simulink model "EKF_InverseDynamic_2dof_pole"  (R2023b)
settings: Solver=VariableStepAuto  StartTime=0.0  StopTime=Tend_slk  RelTol=1e-3
values from neighbouring files (symbols this model uses):
  g = 9.81    [EKF_main_inverse_2dof_pole.m]
  IMU_a_b_bias = ones(3,1)*0.1    [EKF_main_inverse_2dof_pole.m]
  IMU_a_b_variance = IMU_var_bias_matrix(:,1)    [EKF_main_inverse_2dof_pole.m]
  IMU_mf_b_bias = ones(3,1)*0.1    [EKF_main_inverse_2dof_pole.m]
  IMU_mf_b_variance = IMU_var_bias_matrix(:,4)    [EKF_main_inverse_2dof_pole.m]
  IMU_w_b_bias = IMU_var_bias_matrix(:,2)    [EKF_main_inverse_2dof_pole.m]
  IMU_w_b_variance = IMU_var_bias_matrix(:,3)    [EKF_main_inverse_2dof_pole.m]
  mf = [22602; 0; -42062;]    [EKF_main_inverse_2dof_pole.m]
  P0 = diag([P0_ph_meas,P0_th_meas,P0_ps_meas,P0_bias_wp,P0_bias_wq,P0_bias_wr])    [EKF_main_inverse_2dof_pole.m]
  param = [Ixx;Iyy;Izz;l;k1;k2;k3;k4;b;m]    [EKF_main_inverse_2dof_pole.m]
  Q = diag([q_angle,q_angle,q_angle, q_bias_w_b,q_bias_w_b,q_bias_w_b])    [EKF_main_inverse_2dof_pole.m]
  R = diag([r_th_meas,r_th_meas,r_ps_meas])    [EKF_main_inverse_2dof_pole.m]
  Ts_EKF_integr = 0.01    [EKF_main_inverse_2dof_pole.m]
  Ts_EKF_meas = 0.05    [EKF_main_inverse_2dof_pole.m]
  Ts_slk = 0.01    [EKF_main_inverse_2dof_pole.m]
  x0 = [1;1;1;0;0;0]*0.01    [EKF_main_inverse_2dof_pole.m]
  x0EKF = [ph0;th0;ps0;bias_wp0;bias_wq0;bias_wr0]    [EKF_main_inverse_2dof_pole.m]
undefined symbols (not defined in the file or in its folder): Kpole, x_eq
libraries: simulink x3
settings Model: Creator=teoma  LastModifiedBy=asus

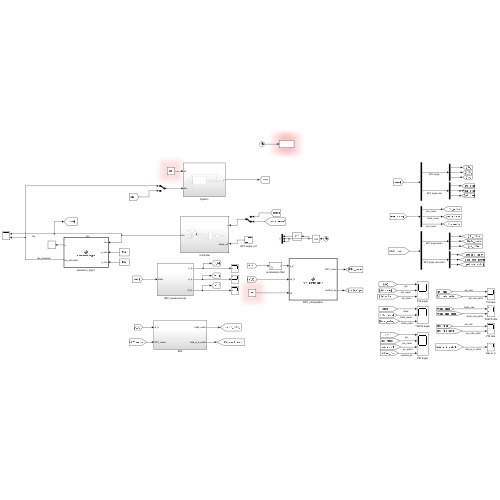
[thumbnail: Simulink's stored preview of the top-level diagram]
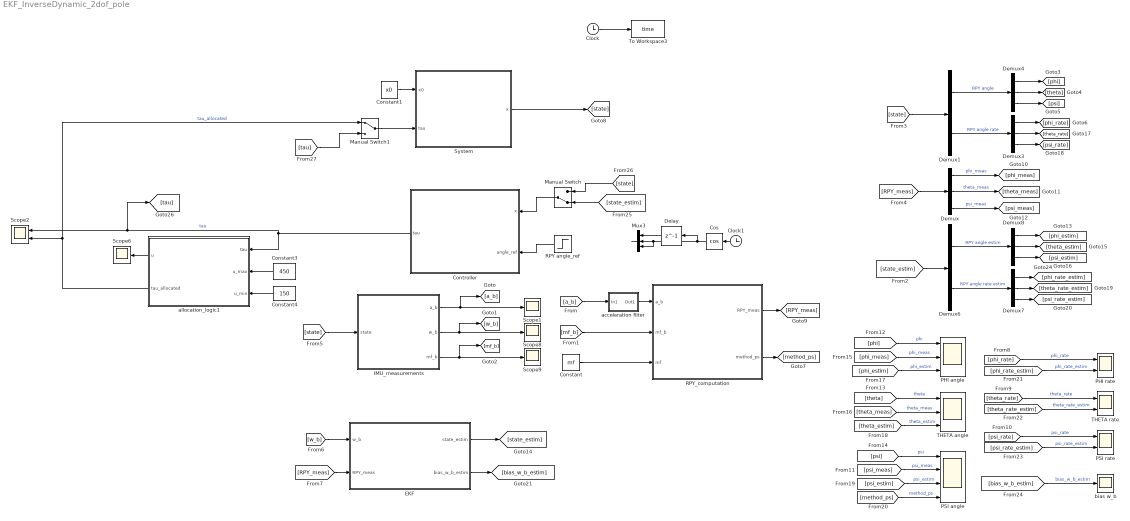
== system EKF_InverseDynamic_2dof_pole ==
  Clock : Clock
  Clock1 : Clock
  Constant : Constant  Value=mf
  Constant1 : Constant  Value=x0
  Constant3 : Constant  Value=450  SampleTime=0.01
  Constant4 : Constant  Value=150  SampleTime=0.01
  Controller : Subsystem
  Cos : Trigonometry  Operator=cos
  Delay : Delay  DelayLength=1  SampleTime=0.01
  Demux{,3..4,7..8} (5 alike) : Demux  Outputs=3
  Demux1 : Demux  Outputs=2
  Demux6 : Demux  Outputs=2
  EKF : Subsystem
  IMU_measurements : Subsystem
  Manual Switch : ManualSwitch  CurrentSetting=0
  Manual Switch1 : ManualSwitch
  Mux3 : Mux  Inputs=3
  PHI angle : Scope  NumInputPorts=3
  PHI rate : Scope  NumInputPorts=2
  PSI angle : Scope  NumInputPorts=4
  PSI rate : Scope  NumInputPorts=2
  RPY angle_ref : Step  Time=20  After=[0.52;0.52]  SampleTime=0
  RPY_computation : MATLAB Function  TreatAsAtomicUnit=on
  Scope{1,6,8..9} (4 alike) : Scope
  Scope2 : Scope  NumInputPorts=2
  System : Subsystem
  THETA angle : Scope  NumInputPorts=3
  THETA rate : Scope  NumInputPorts=2
  To Workspace3 : ToWorkspace  VariableName=time  SampleTime=Ts_slk
      settings: Save2DSignal=2-D array (concatenate along first dimension)
  acceleration filter : Subsystem  mask{p=5}
      mask prompts: p "pole"
  allocation_logic1 : MATLAB Function  TreatAsAtomicUnit=on
  bias w_b : Scope
  wires:
  Demux4/3 -> [psi]
  Demux4/2 -> [theta]
  Constant1/1 -> System/1(x0)
  Demux1/2 -> Demux3/1  "RPY angle rate"
  System/1(x) -> [state]
  Demux4/1 -> [phi]
  Clock/1 -> To Workspace3/1
  Demux1/1 -> Demux4/1  "RPY angle"
  IMU_measurements/1(a_b) -> [a_b], Scope1/1
  IMU_measurements/2(w_b) -> Scope8/1, [w_b]
  IMU_measurements/3(mf_b) -> [mf_b], Scope9/1
  [a_b] -> acceleration filter/1(In1)
  [mf_b] -> RPY_computation/2(mf_b)
  Constant/1 -> RPY_computation/3(mf)
  RPY_computation/1(RPY_meas) -> [RPY_meas]
  [state] -> IMU_measurements/1(state)
  [w_b] -> EKF/1(w_b)
  [RPY_meas] -> EKF/2(RPY_meas)
  [phi] -> PHI angle/1  "phi"
  [phi_meas] -> PHI angle/2  "phi_meas"
  [phi_estim] -> PHI angle/3  "phi_estim"
  [theta] -> THETA angle/1  "theta"
  [theta_meas] -> THETA angle/2  "theta_meas"
  [theta_estim] -> THETA angle/3  "theta_estim"
  [psi] -> PSI angle/1  "psi"
  [psi_meas] -> PSI angle/2  "psi_meas"
  [psi_estim] -> PSI angle/3  "psi_estim"
  RPY_computation/2(method_ps) -> [method_ps]
  acceleration filter/1(Out1) -> RPY_computation/1(a_b)
  EKF/1(state_estim) -> [state_estim]
  EKF/2(bias_w_b_estim) -> [bias_w_b_estim]
  [method_ps] -> PSI angle/4  "method_ps"
  [state] -> Demux1/1
  Demux3/3 -> [psi_rate]
  Demux3/1 -> [phi_rate]
  Demux3/2 -> [theta_rate]
  [RPY_meas] -> Demux/1
  Demux/2 -> [theta_meas]  "theta_meas"
  Demux/3 -> [psi_meas]  "psi_meas"
  Demux/1 -> [phi_meas]  "phi_meas"
  Demux7/1 -> [phi_rate_estim]
  [state_estim] -> Demux6/1
  Demux8/1 -> [phi_estim]
  Demux8/2 -> [theta_estim]
  Demux7/2 -> [theta_rate_estim]
  Demux6/2 -> Demux7/1  "RPY angle rate estim"
  Demux7/3 -> [psi_rate_estim]
  Demux8/3 -> [psi_estim]
  Demux6/1 -> Demux8/1  "RPY angle estim"
  [phi_rate] -> PHI rate/1  "phi_rate"
  [phi_rate_estim] -> PHI rate/2  "phi_rate_estim"
  [psi_rate] -> PSI rate/1  "psi_rate"
  [psi_rate_estim] -> PSI rate/2  "psi_rate_estim"
  [theta_rate] -> THETA rate/1  "theta_rate"
  [theta_rate_estim] -> THETA rate/2  "theta_rate_estim"
  [bias_w_b_estim] -> bias w_b/1  "bias_w_b_estim"
  [state_estim] -> Manual Switch/2
  Clock1/1 -> Cos/1
  Cos/1 -> Mux3/2, Mux3/3, Delay/1
  Delay/1 -> Mux3/1
  Mux3/1 -> ?
  RPY angle_ref/1 -> Controller/2(angle_ref)
  Manual Switch/1 -> Controller/1(x)
  [state] -> Manual Switch/1
  Manual Switch1/1 -> System/2("tau ")
  [tau] -> Manual Switch1/2
  allocation_logic1/1(u) -> Scope6/1
  Controller/1(tau) -> Scope2/1, [tau], allocation_logic1/1(tau)  "tau"
  allocation_logic1/2(tau_allocated) -> Manual Switch1/1, Scope2/2  "tau_allocated"
  Constant3/1 -> allocation_logic1/2(u_max)
  Constant4/1 -> allocation_logic1/3(u_min)

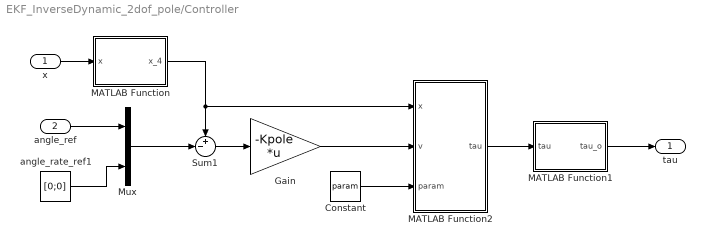
== system EKF_InverseDynamic_2dof_pole/Controller ==
  x : Inport
  angle_ref : Inport  Port=2
  Constant : Constant  Value=param
  Gain : Gain  Gain=-Kpole  Multiplication=Matrix(K*u) (u vector)
  MATLAB Function : MATLAB Function  TreatAsAtomicUnit=on
  MATLAB Function1 : MATLAB Function  TreatAsAtomicUnit=on
  MATLAB Function2 : MATLAB Function  TreatAsAtomicUnit=on
  Mux : Mux  Inputs=2
  Sum1 : Sum  Inputs=+-|
  angle_rate_ref1 : Constant  Value=[0;0]
  tau : Outport
  wires:
  angle_rate_ref1/1 -> Mux/2
  Mux/1 -> Sum1/2
  Constant/1 -> MATLAB Function2/3(param)
  Gain/1 -> MATLAB Function2/2(v)
  MATLAB Function2/1(tau) -> MATLAB Function1/1(tau)
  MATLAB Function/1(x_4) -> MATLAB Function2/1(x), Sum1/1
  angle_ref/1 -> Mux/1
  Sum1/1 -> Gain/1
  MATLAB Function1/1(tau_o) -> tau/1
  x/1 -> MATLAB Function/1(x)

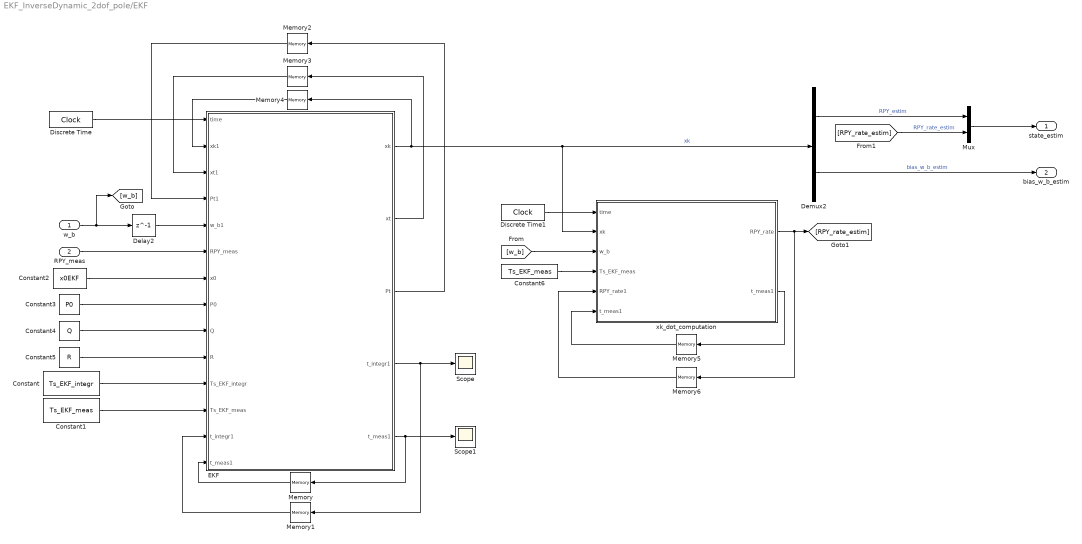
== system EKF_InverseDynamic_2dof_pole/EKF ==
  w_b : Inport
  RPY_meas : Inport  Port=2
  Constant : Constant  Value=Ts_EKF_integr
  Constant1 : Constant  Value=Ts_EKF_meas
  Constant2 : Constant  Value=x0EKF
  Constant3 : Constant  Value=P0
  Constant4 : Constant  Value=Q
  Constant5 : Constant  Value=R
  Constant6 : Constant  Value=Ts_EKF_meas
  Delay2 : Delay  DelayLength=1  SampleTime=Ts_EKF_integr
  Demux2 : Demux  Outputs=2
  Discrete Time : DigitalClock  SampleTime=Ts_slk
  Discrete Time1 : DigitalClock  SampleTime=Ts_slk
  EKF : MATLAB Function  TreatAsAtomicUnit=on
  Memory{,1..6} (7 alike) : Memory
  Mux : Mux  Inputs=2
  Scope : Scope
  Scope1 : Scope
  xk_dot_computation : MATLAB Function  TreatAsAtomicUnit=on
  state_estim : Outport
  bias_w_b_estim : Outport  Port=2
  wires:
  w_b/1 -> Delay2/1, [w_b]
  Constant4/1 -> EKF/9(Q)
  Constant2/1 -> EKF/7(x0)
  Constant5/1 -> EKF/10(R)
  Memory/1 -> EKF/14("t_meas1 ")
  EKF/2(xt) -> Memory3/1
  Memory2/1 -> EKF/4(Pt1)
  EKF/3(Pt) -> Memory2/1
  RPY_meas/1 -> EKF/6(RPY_meas)
  Discrete Time/1 -> EKF/1(time)
  Memory3/1 -> EKF/3(xt1)
  Memory1/1 -> EKF/13("t_integr1 ")
  Constant3/1 -> EKF/8(P0)
  EKF/5(t_meas1) -> Scope1/1, Memory/1
  EKF/4(t_integr1) -> Scope/1, Memory1/1
  Delay2/1 -> EKF/5(w_b1)
  Constant/1 -> EKF/11(Ts_EKF_integr)
  Constant1/1 -> EKF/12(Ts_EKF_meas)
  Memory4/1 -> EKF/2(xk1)
  xk_dot_computation/2(t_meas1) -> Memory5/1
  Memory5/1 -> xk_dot_computation/6("t_meas1 ")
  Memory6/1 -> xk_dot_computation/5(RPY_rate1)
  xk_dot_computation/1(RPY_rate) -> [RPY_rate_estim], Memory6/1
  [w_b] -> xk_dot_computation/3(w_b)
  Discrete Time1/1 -> xk_dot_computation/1(time)
  Demux2/2 -> bias_w_b_estim/1  "bias_w_b_estim"
  Demux2/1 -> Mux/1  "RPY_estim"
  EKF/1(xk) -> xk_dot_computation/2(xk), Demux2/1, Memory4/1  "xk"
  [RPY_rate_estim] -> Mux/2  "RPY_rate_estim"
  Mux/1 -> state_estim/1
  Constant6/1 -> xk_dot_computation/4(Ts_EKF_meas)

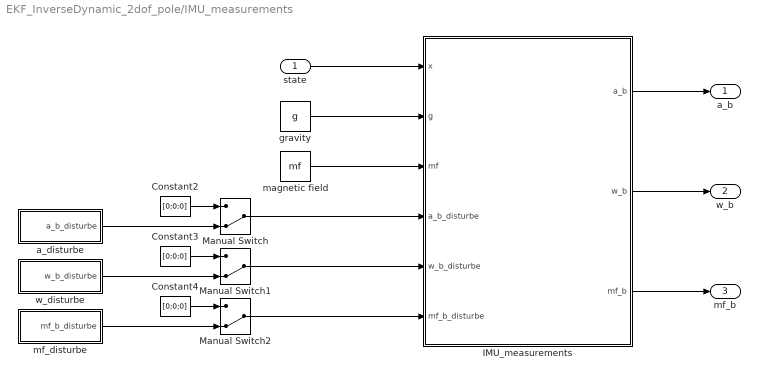
== system EKF_InverseDynamic_2dof_pole/IMU_measurements ==
  state : Inport
  Constant2 : Constant  Value=[0;0;0]
  Constant3 : Constant  Value=[0;0;0]
  Constant4 : Constant  Value=[0;0;0]
  IMU_measurements : MATLAB Function  TreatAsAtomicUnit=on
  Manual Switch : ManualSwitch  CurrentSetting=0
  Manual Switch1 : ManualSwitch  CurrentSetting=0
  Manual Switch2 : ManualSwitch  CurrentSetting=0
  a_disturbe : Subsystem  mask{on_off_bias=on bias, on_off_variance=on variance}
      mask prompts: on_off_bias "on-off bias"; on_off_variance "on-off variance"
  gravity : Constant  Value=g
  magnetic field : Constant  Value=mf
  mf_disturbe : Subsystem  mask{on_off_bias=on bias, on_off_variance=on variance}
      mask prompts: on_off_bias "on-off bias"; on_off_variance "on-off variance"
  w_disturbe : Subsystem  mask{on_off_bias=on bias, on_off_variance=on variance}
      mask prompts: on_off_bias "on-off bias"; on_off_variance "on-off variance"
  a_b : Outport
  w_b : Outport  Port=2
  mf_b : Outport  Port=3
  wires:
  state/1 -> IMU_measurements/1(x)
  gravity/1 -> IMU_measurements/2(g)
  magnetic field/1 -> IMU_measurements/3(mf)
  a_disturbe/1(a_b_disturbe) -> Manual Switch/2
  w_disturbe/1(w_b_disturbe) -> Manual Switch1/2
  mf_disturbe/1(mf_b_disturbe) -> Manual Switch2/2
  IMU_measurements/1(a_b) -> a_b/1
  IMU_measurements/2(w_b) -> w_b/1
  IMU_measurements/3(mf_b) -> mf_b/1
  Constant2/1 -> Manual Switch/1
  Constant3/1 -> Manual Switch1/1
  Constant4/1 -> Manual Switch2/1
  Manual Switch2/1 -> IMU_measurements/6(mf_b_disturbe)
  Manual Switch1/1 -> IMU_measurements/5(w_b_disturbe)
  Manual Switch/1 -> IMU_measurements/4(a_b_disturbe)

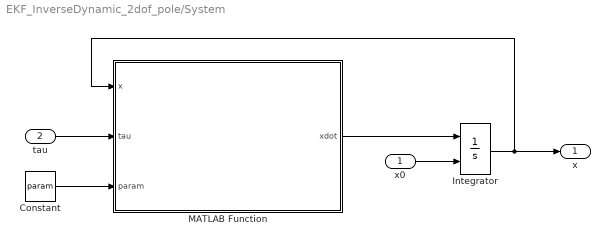
== system EKF_InverseDynamic_2dof_pole/System ==
  x0 : Inport
  "tau " : Inport  Port=2
  Constant : Constant  Value=param
  Integrator : Integrator  InitialConditionSource=external  InitialCondition=x_eq
  MATLAB Function : MATLAB Function  TreatAsAtomicUnit=on
  x : Outport
  wires:
  Integrator/1 -> MATLAB Function/1(x), x/1
  MATLAB Function/1(xdot) -> Integrator/1
  "tau "/1 -> MATLAB Function/2(tau)
  Constant/1 -> MATLAB Function/3(param)
  x0/1 -> Integrator/2

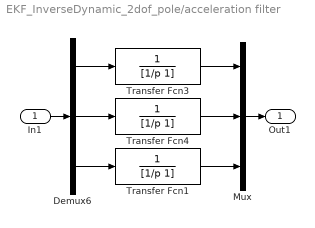
== system EKF_InverseDynamic_2dof_pole/acceleration filter ==
  In1 : Inport
  Demux6 : Demux  Outputs=3
  Mux : Mux  Inputs=3
  Transfer Fcn1 : TransferFcn  Denominator=[1/p 1]
  Transfer Fcn3 : TransferFcn  Denominator=[1/p 1]
  Transfer Fcn4 : TransferFcn  Denominator=[1/p 1]
  Out1 : Outport
  wires:
  Transfer Fcn4/1 -> Mux/2
  Demux6/3 -> Transfer Fcn1/1
  Mux/1 -> Out1/1
  Transfer Fcn1/1 -> Mux/3
  Transfer Fcn3/1 -> Mux/1
  In1/1 -> Demux6/1
  Demux6/1 -> Transfer Fcn3/1
  Demux6/2 -> Transfer Fcn4/1

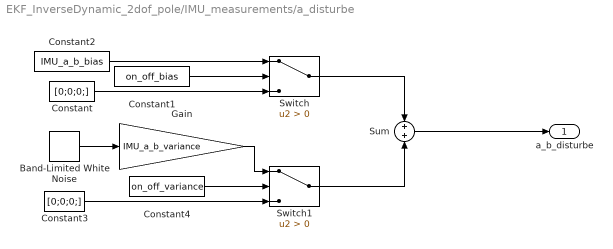
== system EKF_InverseDynamic_2dof_pole/IMU_measurements/a_disturbe ==
  Band-Limited White Noise : simulink/Sources/Band-Limited White Noise  Cov=[1]  Ts=0.1  seed=[23341]
  Constant : Constant  Value=[0;0;0;]
  Constant1 : Constant  Value=on_off_bias
  Constant2 : Constant  Value=IMU_a_b_bias
  Constant3 : Constant  Value=[0;0;0;]
  Constant4 : Constant  Value=on_off_variance
  Gain : Gain  Gain=IMU_a_b_variance
  Sum : Sum  Inputs=+|+
  Switch : Switch  Criteria=u2 > Threshold  SaturateOnIntegerOverflow=off  InputSameDT=off
  Switch1 : Switch  Criteria=u2 > Threshold  SaturateOnIntegerOverflow=off  InputSameDT=off
  a_b_disturbe : Outport
  wires:
  Constant2/1 -> Switch/1
  Sum/1 -> a_b_disturbe/1
  Constant/1 -> Switch/3
  Constant1/1 -> Switch/2
  Band-Limited White Noise/1 -> Gain/1
  Gain/1 -> Switch1/1
  Constant3/1 -> Switch1/3
  Constant4/1 -> Switch1/2
  Switch/1 -> Sum/1
  Switch1/1 -> Sum/2

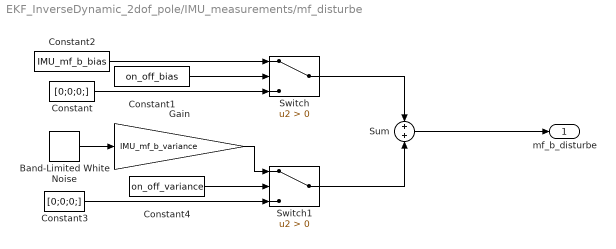
== system EKF_InverseDynamic_2dof_pole/IMU_measurements/mf_disturbe ==
  Band-Limited White Noise : simulink/Sources/Band-Limited White Noise  Cov=[1]  Ts=0.1  seed=[23341]
  Constant : Constant  Value=[0;0;0;]
  Constant1 : Constant  Value=on_off_bias
  Constant2 : Constant  Value=IMU_mf_b_bias
  Constant3 : Constant  Value=[0;0;0;]
  Constant4 : Constant  Value=on_off_variance
  Gain : Gain  Gain=IMU_mf_b_variance
  Sum : Sum  Inputs=+|+
  Switch : Switch  Criteria=u2 > Threshold  SaturateOnIntegerOverflow=off  InputSameDT=off
  Switch1 : Switch  Criteria=u2 > Threshold  SaturateOnIntegerOverflow=off  InputSameDT=off
  mf_b_disturbe : Outport
  wires:
  Constant2/1 -> Switch/1
  Sum/1 -> mf_b_disturbe/1
  Constant/1 -> Switch/3
  Constant1/1 -> Switch/2
  Band-Limited White Noise/1 -> Gain/1
  Gain/1 -> Switch1/1
  Constant3/1 -> Switch1/3
  Constant4/1 -> Switch1/2
  Switch/1 -> Sum/1
  Switch1/1 -> Sum/2

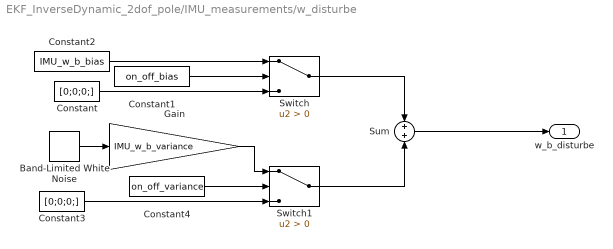
== system EKF_InverseDynamic_2dof_pole/IMU_measurements/w_disturbe ==
  Band-Limited White Noise : simulink/Sources/Band-Limited White Noise  Cov=[1]  Ts=0.1  seed=[23341]
  Constant : Constant  Value=[0;0;0;]
  Constant1 : Constant  Value=on_off_bias
  Constant2 : Constant  Value=IMU_w_b_bias
  Constant3 : Constant  Value=[0;0;0;]
  Constant4 : Constant  Value=on_off_variance
  Gain : Gain  Gain=IMU_w_b_variance
  Sum : Sum  Inputs=+|+
  Switch : Switch  Criteria=u2 > Threshold  SaturateOnIntegerOverflow=off  InputSameDT=off
  Switch1 : Switch  Criteria=u2 > Threshold  SaturateOnIntegerOverflow=off  InputSameDT=off
  w_b_disturbe : Outport
  wires:
  Constant2/1 -> Switch/1
  Sum/1 -> w_b_disturbe/1
  Constant/1 -> Switch/3
  Constant1/1 -> Switch/2
  Band-Limited White Noise/1 -> Gain/1
  Gain/1 -> Switch1/1
  Constant3/1 -> Switch1/3
  Constant4/1 -> Switch1/2
  Switch/1 -> Sum/1
  Switch1/1 -> Sum/2

== matlab function EKF_InverseDynamic_2dof_pole/Controller/MATLAB Function1 ==
  data: tau input; tau_o output
function tau_o=fcn(tau)
% Inputs:   tau    (torque 2x1)         
%
% Outputs:  tau_o  (torque 3x1)

% States in input
tau_1     =       tau(1,1);     %  roll torque
tau_2     =       tau(2,1);     %  pitch torque
 


% States in output
tau_o      =       zeros(3,1);
tau_o(1,1) =       tau_1;   
tau_o(2,1) =       tau_2;
tau_o(3,1) =       0;

== matlab function EKF_InverseDynamic_2dof_pole/Controller/MATLAB Function2 ==
  data: x input; v input; tau output; param input
function tau = fcn(x,v,param)
% Inputs:
%           x       (model state)
%           v       (new input to the feedback system)           
%           param   (model parameters)
%
% Outputs:  tau     (torque)

% Parameters
g        =       9.81;           %  gravity acceleration (m/s^2)
Ixx      =       param(1,1);     %  moment of inertia 
Iyy      =       param(2,1);     %  moment of inertia
Izz      =       param(3,1);     %  moment of inertia 

% States
phi      =       x(1,1);     %  roll angle (rad)
theta    =       x(2,1);     %  pitch angle (rad)
phi_dot  =       x(3,1);     %  roll rate (rad/s)
theta_dot=       x(4,1);     %  pitch rate (rad/s)

cph         =       cos(phi);
cth         =       cos(theta);
sph         =       sin(phi);
sth         =       sin(theta);

% Coriolis matrix
C11=  0;
C12= (Iyy)*(theta_dot*cph*sph);
C21= (Iyy)*(theta_dot*cph*sph);
C22= 0;

C  = [C11 C12;
      C21 C22];

% Inertia matrix
J11= Ixx;
J12= 0;
J21= 0;
J22= Iyy*cph^2;

J  = [J11 J12;
     J21 J22];

%% Control law
tau = zeros(2,1);
tau = J*v+C*x(3:4,1);

== matlab function EKF_InverseDynamic_2dof_pole/allocation_logic1 ==
  data: tau input; u_max input; u output; tau_allocated output; u_min input; param parameter
function [u, tau_allocated] = allocation_logic(tau,u_max,u_min,param)
% Allocation Logic Block: computes the corresponding control command
% u = [u1,u2,u3,u4] given the torque command tau = [tau_phi, tau_theta, tau_phi]

% control command limits
%%u_min = 100;
% u_max = 1000;

l  = param(4,1);
k1 = param(5,1);
k2 = param(6,1);
k3 = param(7,1);
k4 = param(8,1);
b  = param(9,1);

u = zeros(4,1);
% [tau_ph; tau_th; tau_ps] = Mtau_u * [u1;u2;u3;u4]
Mtau_u = [0       0        l*k3    -l*k4;
         -l*k1    l*k2     0        0;
         -b      -b        b        b;];
% Minv = Mtau_u'*inv(Mtau_u*Mtau_u');
% up = Minv*tau;
% un = zeros(4,1);
% if min(up(:)) < u_min 
%     un = ones(4,1)*(u_min - min(up(:)));
% end
% u = up+un;
% for i = 1:1:4
%     if u(i,1) > u_max
%         u(i,1) = u_max;
%     end
% end
if tau(1) >= 0
    u(4) = u_min;
    u(3) = (tau(1) + l*k4*u(4))/(l*k3);
else
    u(3) = u_min;
    u(4) = (-tau(1) + l*k3*u(3))/(l*k4);
end
if tau(2) >= 0
    u(1) = u_min;
    u(2) = (tau(2) + l*k1*u(1))/(l*k2);
else
    u(2) = u_min;
    u(1) = (-tau(2) + l*k2*u(2))/(l*k1);
end
u = min(u_max,u);
tau_allocated = Mtau_u*u;

== matlab function EKF_InverseDynamic_2dof_pole/Controller/MATLAB Function ==
  data: x input; x_4 output
function x_4=fcn(x)
% Inputs:   x      (model state 6x1)         
%
% Outputs:  x_4  (model state 4x1)

% States in input
phi      =       x(1,1);     %  roll angle (rad)
theta    =       x(2,1);     %  pitch angle (rad)
psi      =       x(3,1);     %  yaw angle (rad)  
phi_dot  =       x(4,1);     %  roll rate (rad/s)
theta_dot=       x(5,1);     %  pitch rate (rad/s)
psi_dot  =       x(6,1);     %  yaw rate (rad/s)  


% States in output
x_4      =       zeros(4,1);
x_4(1,1) =       phi;   
x_4(2,1) =       theta;
x_4(3,1) =       phi_dot;
x_4(4,1) =       theta_dot;

== matlab function EKF_InverseDynamic_2dof_pole/System/MATLAB Function ==
  data: x input; tau input; xdot output; param input
function xdot=quadcopter(x,tau,param)
% Inputs:
%           x       (model state)
%           tau     (torque)           
%           param   (model parameters)
%
% Outputs:  x_dot  (derivative of the state with respect to time)

% Parameters
g        =       9.81;           %  gravity acceleration (m/s^2)
Ixx      =       param(1,1);     %  moment of inertia 
Iyy      =       param(2,1);     %  moment of inertia
Izz      =       param(3,1);     %  moment of inertia 

% States
phi      =       x(1,1);     %  roll angle (rad)
theta    =       x(2,1);     %  pitch angle (rad)
psi      =       x(3,1);     %  yaw angle (rad)  
phi_dot  =       x(4,1);     %  roll rate (rad/s)
theta_dot=       x(5,1);     %  pitch rate (rad/s)
psi_dot  =       x(6,1);     %  yaw rate (rad/s)  

cph         =       cos(phi);
cth         =       cos(theta);
cps         =       cos(psi);
sph         =       sin(phi);
sth         =       sin(theta);
sps         =       sin(psi);  

% Coriolis matrix
C11=  0;
C12= (Iyy-Izz)*(theta_dot*cph*sph+psi_dot*sph^2*cth)+(Izz-Iyy)*psi_dot*cph^2*cth-Ixx*psi_dot*cth;
C13= (Izz-Iyy)*psi_dot*cph*sph*cth^2;
C21= (Izz-Iyy)*(theta_dot*cph*sph+psi_dot*sph*cth)+(Iyy-Izz)*psi_dot*cph^2*cth+Ixx*psi_dot*cth;
C22= (Izz-Iyy)*psi_dot*cph*sph;
C23= -Ixx*psi_dot*sth*cth+Iyy*psi_dot*sph^2*sth*cth+Izz*psi_dot*cph^2*sth*cth;
C31= (Iyy-Izz)*psi_dot*cth^2*sph*cph-Ixx*theta_dot*cth;
C32= (Izz-Iyy)*(theta_dot*cph*sph*sth+phi_dot*sph^2*cth)+(Iyy-Izz)*phi_dot*cph^2*cth+Ixx*psi_dot*sth*cth-Iyy*psi_dot*sph^2*sth*cth-Izz*psi_dot*cph^2*sth*cth;
C33= (Iyy-Izz)*phi_dot*cph*sph*cth^2-Iyy*theta_dot*sph^2*cth*sth-Izz*theta_dot*cph^2*cth*sth+Ixx*theta_dot*cth*sth;

C  = [C11 C12 C13;
    C21 C22 C23;
    C31 C32 C33];

% Inertia matrix
J11= Ixx;
J12= 0;
J13= -Ixx*sth;
J21= 0;
J22= Iyy*cph^2+Izz*sph^2;
J23= (Iyy-Izz)*cph*sph*cth;
J31= -Ixx*sth;
J32= (Iyy-Izz)*cph*sph*cth;
J33= Ixx*sth^2+Iyy*sph^2*cth^2+Izz*cph^2*cth^2;

J  = [J11 J12 J13;
    J21 J22 J23;
    J31 J32 J33];
%% Model equations
invJ = [ (J22*J33 - J23*J32)/(J11*J22*J33 - J11*J23*J32 - J12*J21*J33 + J12*J23*J31 + J13*J21*J32 - J13*J22*J31), -(J12*J33 - J13*J32)/(J11*J22*J33 - J11*J23*J32 - J12*J21*J33 + J12*J23*J31 + J13*J21*J32 - J13*J22*J31),  (J12*J23 - J13*J22)/(J11*J22*J33 - J11*J23*J32 - J12*J21*J33 + J12*J23*J31 + J13*J21*J32 - J13*J22*J31);
         -(J21*J33 - J23*J31)/(J11*J22*J33 - J11*J23*J32 - J12*J21*J33 + J12*J23*J31 + J13*J21*J32 - J13*J22*J31),  (J11*J33 - J13*J31)/(J11*J22*J33 - J11*J23*J32 - J12*J21*J33 + J12*J23*J31 + J13*J21*J32 - J13*J22*J31), -(J11*J23 - J13*J21)/(J11*J22*J33 - J11*J23*J32 - J12*J21*J33 + J12*J23*J31 + J13*J21*J32 - J13*J22*J31);
         (J21*J32 - J22*J31)/(J11*J22*J33 - J11*J23*J32 - J12*J21*J33 + J12*J23*J31 + J13*J21*J32 - J13*J22*J31), -(J11*J32 - J12*J31)/(J11*J22*J33 - J11*J23*J32 - J12*J21*J33 + J12*J23*J31 + J13*J21*J32 - J13*J22*J31),  (J11*J22 - J12*J21)/(J11*J22*J33 - J11*J23*J32 - J12*J21*J33 + J12*J23*J31 + J13*J21*J32 - J13*J22*J31);];

xdot        = zeros(6,1);
xdot(1:3,1) = x(4:6,1);
xdot(4:6,1) = invJ*(tau - C*x(4:6,1));

== matlab function EKF_InverseDynamic_2dof_pole/IMU_measurements/IMU_measurements ==
  data: x input; a_b output; g input; mf input; a_b_disturbe input; w_b_disturbe input; mf_b_disturbe input; w_b output; mf_b output
function [a_b, w_b, mf_b] = IMU_measurements(x,g,mf,a_b_disturbe,w_b_disturbe,mf_b_disturbe)
% description:
% - a_b             = measured linear acceleration in body-frame
% - w_b             = measured angular velocity in body-frame
% - mf_b            = measured magnetic field in body-frame
% - a_b_disturbe    = linear velocity measurement-noise
% - w_b_disturbe    = angular velocity measurement-noise
% - mf_b_disturbe   = magnetic field measurement-noise

% States
phi      =       x(1,1);     %  roll angle (rad)
theta    =       x(2,1);     %  pitch angle (rad)
psi      =       x(3,1);     %  yaw angle (rad)  
phi_dot  =       x(4,1);     %  roll rate (rad/s)
theta_dot=       x(5,1);     %  pitch rate (rad/s)
psi_dot  =       x(6,1);     %  yaw rate (rad/s)  

cph         =       cos(phi);
cth         =       cos(theta);
cps         =       cos(psi);
sph         =       sin(phi);
sth         =       sin(theta);
sps         =       sin(psi);  


% acceleration
a_b = -g*[-sth;sph*cth;cph*cth] + a_b_disturbe;

% angular velocity
Wn = [1,        0,      -sth;
      0,        cph,    cth*sph;
      0,        -sph,   cth*cph;];
w_b = Wn*[phi_dot;theta_dot;psi_dot] + w_b_disturbe;

% magnetic field
R = [cps*cth,                0,  -sth;
     cps*sth*sph-sps*cph,    0,  cth*sph;
     cps*sth*cph+sps*sph,    0,  cth*cph;];
mf_b = R*mf + mf_b_disturbe;

== matlab function EKF_InverseDynamic_2dof_pole/RPY_computation ==
  data: a_b input; mf_b input; RPY_meas output; mf input; method_ps output
function [RPY_meas,method_ps]   = RPY_computation(a_b,mf_b,mf)
% description:
% - a_b             = measured linear acceleration in body-frame
% - w_b             = measured angular velocity in body-frame
% - mf_b            = measured magnetic field in body-frame
% - mf              = measured magnetic field in body-inertia
% - a_b_disturbe    = linear velocity measurement-noise
% - w_b_disturbe    = angular velocity measurement-noise
% - mf_b_disturbe   = magnetic field measurement-noise

% -------------------------------------------------------------------------------------------
% observation: the following computation works only if the angles
% phi,theta,psy are withing angles (-pi/2,+pi/2) (this is an open set, pi/2 is excluded)
% -------------------------------------------------------------------------------------------

a_b = -1*a_b;       % need to adjust the sign to use atan2() function correctly
mf_u = mf(3,1);     % magnetic field in up direction (z-dir in inertia frame)

% phi computation
ph_meas = atan2(a_b(2), a_b(3));
sph = sin(ph_meas);
cph = cos(ph_meas);

% theta computation
th_meas = atan2(-a_b(1), (a_b(2)*sph + a_b(3)*cph));
sth = sin(th_meas);
cth = cos(th_meas);

% psi computation
if abs(sin(th_meas)) > 0.1  % sin(th) != 0 
    method_ps = 1;
    ps_meas_numerator   = (sth*cph*mf_b(2) - sth*sph*mf_b(3))/(-sth);       % don't modify
    ps_meas_denominator = (-sph*mf_b(2) - cph*mf_b(3) + cth*mf_u)/(-sth);   % don't modify
    ps_meas = atan2(ps_meas_numerator, ps_meas_denominator);
else                        % sin(th) == 0
    method_ps = 2;
    ps_meas_numerator   = (mf_b(2) - cth*sph*mf_u)*(-cth);
    ps_meas_denominator = cph*mf_b(1);
    ps_meas = atan2(ps_meas_numerator, ps_meas_denominator);
end
RPY_meas = [ph_meas;th_meas;ps_meas];

== matlab function EKF_InverseDynamic_2dof_pole/EKF/EKF ==
  data: time input; xk1 input; xt1 input; Pt1 input; w_b1 input; RPY_meas input; x0 input; P0 input; Q input; R input; Ts_EKF_integr input; Ts_EKF_meas input; xk output; t_integr1 input; t_meas1 input; xt output; Pt output; t_integr1 output; t_meas1 output
function [xk,xt,Pt,t_integr1,t_meas1] = EKF(time,xk1,xt1,Pt1,w_b1,RPY_meas,x0,P0,Q,R,Ts_EKF_integr,Ts_EKF_meas,t_integr1,t_meas1)

if time == 0
    xk = x0;
    xt = x0;
    Pt = P0;
    t_integr1 = 0;
    t_meas1 = 0;
elseif time - t_integr1 >= Ts_EKF_integr
    wp          =       w_b1(1,1);        % p-dir of angular velocity w
    wq          =       w_b1(2,1);        % q-dir of angular velocity w
    wr          =       w_b1(3,1);        % r-dir of angular velocity w

    phi         =       xt1(1,1);         %  roll angle (rad)
    theta       =       xt1(2,1);         %  pitch angle (rad)
    psi         =       xt1(3,1);         %  yaw angle (rad)  
    bias_wp     =       xt1(4,1);         % bias of p-dir of angular velocity w
    bias_wq     =       xt1(5,1);         % bias of q-dir of angular velocity w
    bias_wr     =       xt1(6,1);         % bias of r-dir of angular velocity w

    cph         =       cos(phi);
    cth         =       cos(theta);
    cps         =       cos(psi);
    sph         =       sin(phi);
    sth         =       sin(theta);
    sps         =       sin(psi);
    tth         =       sth/cth;

    % integration step
    t_integr1 = time;
    Mf = [1,    sph*tth,    cph*tth,    0,  0,  0;
          0,    cph,        -sph,       0,  0,  0;
          0,    sph/cth,    cph/cth,    0,  0,  0;
          0,    0,          0,          1,  0,  0;
          0,    0,          0,          0,  1,  0;
          0,    0,          0,          0,  0,  1;];
    Z1 = [wp-bias_wp; wq-bias_wq; wr-bias_wr; bias_wp; bias_wq; bias_wr;];
    f = Mf*Z1;
    xt = xt1 + Ts_EKF_integr*f;

    A1 = [cph*tth*(wq-bias_wq)-sph*tth*(wr-bias_wr),(sph*(wq-bias_wq)+cph*(wr-bias_wr))/cth^2,  0,  -1, -sph*tth,   -cph*tth;];
    A2 = [-sph*(wq-bias_wq)-cph*(wr-bias_wr),   0,  0,  0,  -cph,   sph;];
    A3 = [cph*(wq-bias_wq)/cth-sph*(wr-bias_wr)/cth, (sth/cth^2)*(sph*(wq-bias_wq)+cph*(wr-bias_wr)),   0,  0,  -sph/cth,   -cph/cth;];
    A4 = [0,    0,  0,  1,  0,  0;];
    A5 = [0,    0,  0,  0,  1,  0;];
    A6 = [0,    0,  0,  0,  0,  1;];
    At1 = [A1; A2; A3; A4; A5; A6;];
    Pt = Pt1 + Ts_EKF_integr*(At1*Pt1 + Pt1*At1' + Q);

    % measurement step
    if time - t_meas1 >= Ts_EKF_meas
        t_meas1 = time;
        Ck = [eye(3),zeros(3,3)];
        Lk = Pt*Ck'/(Ck*Pt*Ck' + R);
        xk = xt + Lk*(RPY_meas - Ck*xt);
        Pk = (eye(6) - Lk*Ck)*Pt;

        xt = xk;    % becomes the new xt1
        Pt = Pk;    % becomes the new Pt1
    else
        xk = xk1;    % xk1
    end
else
    xk = xt1;
    xt = xt1;
    Pt = Pt1;
end
end

== matlab function EKF_InverseDynamic_2dof_pole/EKF/xk_dot_computation ==
  data: time input; xk input; w_b input; Ts_EKF_meas input; RPY_rate1 input; RPY_rate output; t_meas1 input; t_meas1 output
function [RPY_rate,t_meas1] = xk_dot_computation(time,xk,w_b,Ts_EKF_meas,RPY_rate1,t_meas1)
RPY_rate = zeros(3,1);
if time == 0
    t_meas1 = 0;
end
if time - t_meas1 >= Ts_EKF_meas || time == 0
    wp          =       w_b(1,1);        % p-dir of angular velocity w
    wq          =       w_b(2,1);        % q-dir of angular velocity w
    wr          =       w_b(3,1);        % r-dir of angular velocity w

    phi         =       xk(1,1);         %  roll angle (rad)
    theta       =       xk(2,1);         %  pitch angle (rad)
    psi         =       xk(3,1);         %  yaw angle (rad)  
    bias_wp     =       xk(4,1)*0;         % bias of p-dir of angular velocity w
    bias_wq     =       xk(5,1)*0;         % bias of q-dir of angular velocity w
    bias_wr     =       xk(6,1)*0;         % bias of r-dir of angular velocity w

    cph         =       cos(phi);
    cth         =       cos(theta);
    cps         =       cos(psi);
    sph         =       sin(phi);
    sth         =       sin(theta);
    sps         =       sin(psi);
    tth         =       sth/cth;

    % integration step
    t_meas1 = time;
    W_eta = [1,    sph*tth,    cph*tth;
             0,    cph,        -sph;
             0,    sph/cth,    cph/cth;];
    w_b_corrected = [wp-bias_wp; wq-bias_wq; wr-bias_wr;];
    RPY_rate = W_eta*w_b_corrected;
else
    RPY_rate = RPY_rate1;
end
end
